simulink model "MovTra"  (R2023b)
settings: Solver=VariableStepAuto  StartTime=0.0  StopTime=15  RelTol=1e-3
values from neighbouring files (symbols this model uses):
  b1 = 1000    [MTvariables.mat]    (also in MovTraslacional.m)
  f = 0    [MTvariables.mat]    (also in MovTraslacional.m)
  k1 = 16182    [MTvariables.mat]    (also in MovTraslacional.m)
  k2 = 19000    [MTvariables.mat]    (also in MovTraslacional.m)
  m1 = 290    [MTvariables.mat]    (also in MovTraslacional.m)
  m2 = 59    [MTvariables.mat]    (also in MovTraslacional.m)

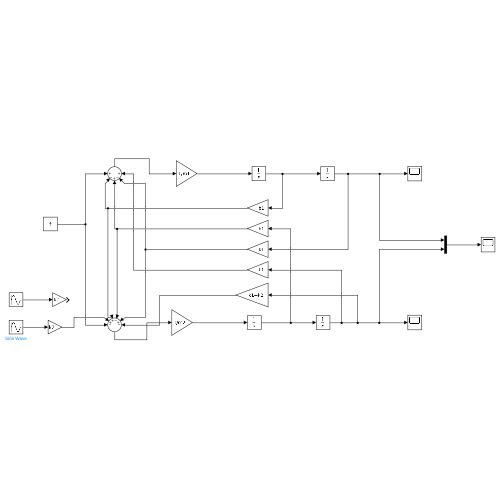
[thumbnail: Simulink's stored preview of the top-level diagram]
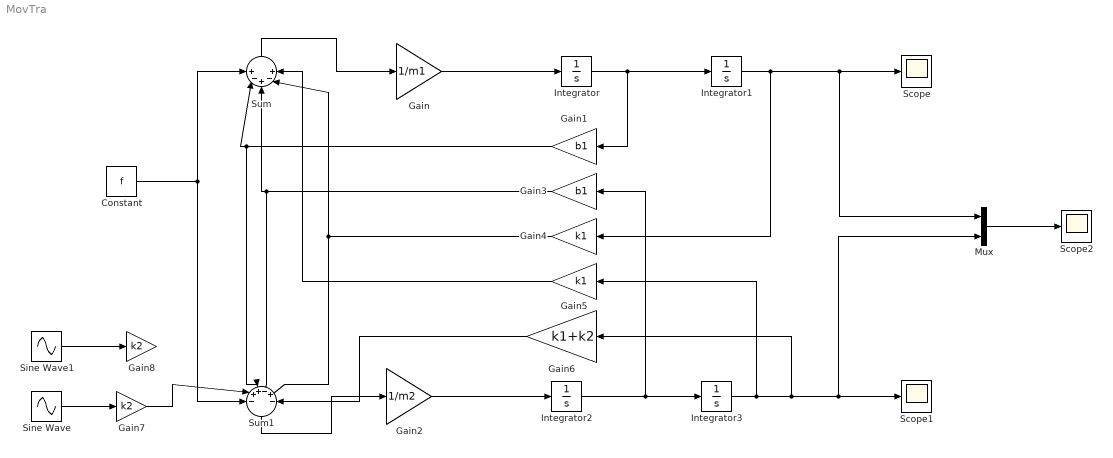
== system MovTra ==
  Constant : Constant  Value=f
  Gain : Gain  Gain=1/m1
  Gain1 : Gain  Gain=b1
  Gain2 : Gain  Gain=1/m2
  Gain3 : Gain  Gain=b1
  Gain4 : Gain  Gain=k1
  Gain5 : Gain  Gain=k1
  Gain6 : Gain  Gain=k1+k2
  Gain7 : Gain  Gain=k2
  Gain8 : Gain  Gain=k2
  Integrator{,1..3} (4 alike) : Integrator
  Mux : Mux  Inputs=2
  Scope : Scope
  Scope1 : Scope
  Scope2 : Scope
  Sine Wave : Sin  Amplitude=0.05  Frequency=0.5*pi  SampleTime=0
  Sine Wave1 : Sin  Amplitude=0.05  Frequency=20*pi  SampleTime=0
  Sum : Sum  Inputs=+-+-+
  Sum1 : Sum  Inputs=-++-+-
  wires:
  Integrator/1 -> Gain1/1, Integrator1/1
  Gain/1 -> Integrator/1
  Sum/1 -> Gain/1
  Integrator2/1 -> Gain3/1, Integrator3/1
  Gain2/1 -> Integrator2/1
  Sum1/1 -> Gain2/1
  Integrator1/1 -> Mux/1, Scope/1, Gain4/1
  Integrator3/1 -> Gain5/1, Gain6/1, Mux/2, Scope1/1
  Gain1/1 -> Sum/2, Sum1/3
  Gain3/1 -> Sum1/4, Sum/3
  Gain4/1 -> Sum1/5, Sum/4
  Gain5/1 -> Sum/5
  Constant/1 -> Sum1/1, Sum/1
  Mux/1 -> Scope2/1
  Sine Wave/1 -> Gain7/1
  Gain6/1 -> Sum1/6
  Sine Wave1/1 -> Gain8/1
  Gain7/1 -> Sum1/2
